simulink model "q2_sim_pid"  (R2019b)
settings: Solver=VariableStepAuto  StartTime=0.0  StopTime=50  RelTol=1e-3
libraries: simulink x2
settings Model: Creator=Mertcan  LastModifiedBy=Mertcan

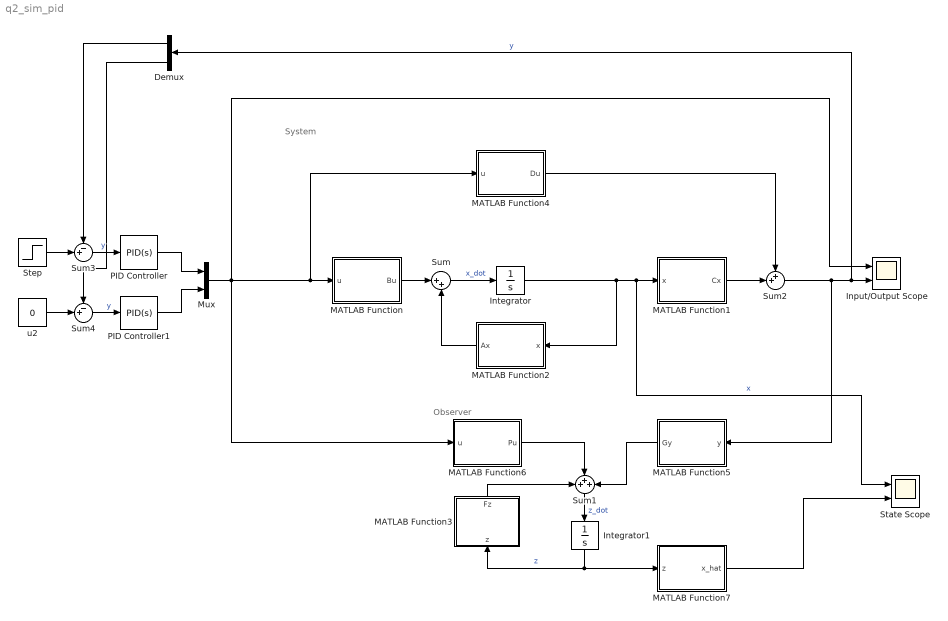
== system q2_sim_pid ==
  note: Observer
  note: System
  Demux : Demux  Outputs=2
  Input/Output Scope : Scope  NumInputPorts=2
  Integrator : Integrator
  Integrator1 : Integrator
  MATLAB Function : MATLAB Function  TreatAsAtomicUnit=on
  MATLAB Function1 : MATLAB Function  TreatAsAtomicUnit=on
  MATLAB Function2 : MATLAB Function  TreatAsAtomicUnit=on
  MATLAB Function3 : MATLAB Function  TreatAsAtomicUnit=on
  MATLAB Function4 : MATLAB Function  TreatAsAtomicUnit=on
  MATLAB Function5 : MATLAB Function  TreatAsAtomicUnit=on
  MATLAB Function6 : MATLAB Function  TreatAsAtomicUnit=on
  MATLAB Function7 : MATLAB Function  TreatAsAtomicUnit=on
  Mux : Mux  Inputs=2
  PID Controller : simulink/Continuous/PID Controller  Controller=PID  Form=Parallel  TimeDomain=Continuous-time  SampleTime=-1  IntegratorMethod=Forward Euler  FilterMethod=Forward Euler  ControllerParametersSource=internal  P=1  I=1  D=0  UseFilter=on  N=100  TunerSelectOption=Transfer Function Based (PID Tuner App)  InitialConditionSource=internal  InitialConditionForIntegrator=0  InitialConditionForFilter=0  DifferentiatorICPrevScaledInput=0  ExternalReset=none  TrackingMode=off  Kt=1  LimitOutput=off  UpperSaturationLimit=inf  LowerSaturationLimit=-inf  LinearizeAsGain=on  AntiWindupMode=none  Kb=1  POutMin=[]  POutMax=[]  IOutMin=[]  IOutMax=[]  DOutMin=[]  DOutMax=[]  NOutMin=[]  NOutMax=[]  SumOutMin=[]  SumOutMax=[]  SaturationOutMin=[]  SaturationOutMax=[]  PParamMin=[]  PParamMax=[]  IParamMin=[]  IParamMax=[]  DParamMin=[]  DParamMax=[]  NParamMin=[]  NParamMax=[]  KbParamMin=[]  KbParamMax=[]  KtParamMin=[]  KtParamMax=[]  KbOutMin=[]  KbOutMax=[]  KtOutMin=[]  KtOutMax=[]  IntegratorOutMin=[]  IntegratorOutMax=[]  FilterOutMin=[]  FilterOutMax=[]  SumI1OutMin=[]  SumI1OutMax=[]  SumI2OutMin=[]  SumI2OutMax=[]  SumI3OutMin=[]  SumI3OutMax=[]  SumI4OutMin=[]  SumI4OutMax=[]  SumDOutMin=[]  SumDOutMax=[]  DifferentiatorOutMin=[]  DifferentiatorOutMax=[]  FilterDiffOutCoefMin=[]  FilterDiffOutCoefMax=[]  ReciprocalOutMin=[]  ReciprocalOutMax=[]  SumDenOutMin=[]  SumDenOutMax=[]  SumNumOutMin=[]  SumNumOutMax=[]  DivideOutMin=[]  DivideOutMax=[]  IntegratorContinuousStateAttributes=''  IntegratorStateMustResolveToSignalObject=off  IntegratorRTWStateStorageClass=Auto  FilterContinuousStateAttributes=''  FilterStateMustResolveToSignalObject=off  FilterRTWStateStorageClass=Auto  ParallelPVariant=InternalParameters  IdealPVariant=Disabled  IVariant=InternalParameters  DVariant=InternalParameters  IntegratorVariant=Continuous  SatVariant=Disabled  AWVariant=Passthrough  PCopyVariant=Disabled  TRVariant=Disabled  FdbkBlocksVariant=Forward  IdealPFdbkVariant=Disabled  SatFdbkVariant=Disabled  DerivativeFilterVariant=ContFilter  NVariant=InternalParameters  NCopyVariant=Disabled  FilterICVariant=InternalICsFilter  IntegratorICVariant=InternalICs  ExternalResetVariant=Disabled  TRSumVariant=Passthrough  SumFdbkVariant=Disabled  SumVariant=Sum_PID
  PID Controller1 : simulink/Continuous/PID Controller  Controller=PID  Form=Parallel  TimeDomain=Continuous-time  SampleTime=-1  IntegratorMethod=Forward Euler  FilterMethod=Forward Euler  ControllerParametersSource=internal  P=1  I=1  D=0  UseFilter=on  N=100  TunerSelectOption=Transfer Function Based (PID Tuner App)  InitialConditionSource=internal  InitialConditionForIntegrator=0  InitialConditionForFilter=0  DifferentiatorICPrevScaledInput=0  ExternalReset=none  TrackingMode=off  Kt=1  LimitOutput=off  UpperSaturationLimit=inf  LowerSaturationLimit=-inf  LinearizeAsGain=on  AntiWindupMode=none  Kb=1  POutMin=[]  POutMax=[]  IOutMin=[]  IOutMax=[]  DOutMin=[]  DOutMax=[]  NOutMin=[]  NOutMax=[]  SumOutMin=[]  SumOutMax=[]  SaturationOutMin=[]  SaturationOutMax=[]  PParamMin=[]  PParamMax=[]  IParamMin=[]  IParamMax=[]  DParamMin=[]  DParamMax=[]  NParamMin=[]  NParamMax=[]  KbParamMin=[]  KbParamMax=[]  KtParamMin=[]  KtParamMax=[]  KbOutMin=[]  KbOutMax=[]  KtOutMin=[]  KtOutMax=[]  IntegratorOutMin=[]  IntegratorOutMax=[]  FilterOutMin=[]  FilterOutMax=[]  SumI1OutMin=[]  SumI1OutMax=[]  SumI2OutMin=[]  SumI2OutMax=[]  SumI3OutMin=[]  SumI3OutMax=[]  SumI4OutMin=[]  SumI4OutMax=[]  SumDOutMin=[]  SumDOutMax=[]  DifferentiatorOutMin=[]  DifferentiatorOutMax=[]  FilterDiffOutCoefMin=[]  FilterDiffOutCoefMax=[]  ReciprocalOutMin=[]  ReciprocalOutMax=[]  SumDenOutMin=[]  SumDenOutMax=[]  SumNumOutMin=[]  SumNumOutMax=[]  DivideOutMin=[]  DivideOutMax=[]  IntegratorContinuousStateAttributes=''  IntegratorStateMustResolveToSignalObject=off  IntegratorRTWStateStorageClass=Auto  FilterContinuousStateAttributes=''  FilterStateMustResolveToSignalObject=off  FilterRTWStateStorageClass=Auto  ParallelPVariant=InternalParameters  IdealPVariant=Disabled  IVariant=InternalParameters  DVariant=InternalParameters  IntegratorVariant=Continuous  SatVariant=Disabled  AWVariant=Passthrough  PCopyVariant=Disabled  TRVariant=Disabled  FdbkBlocksVariant=Forward  IdealPFdbkVariant=Disabled  SatFdbkVariant=Disabled  DerivativeFilterVariant=ContFilter  NVariant=InternalParameters  NCopyVariant=Disabled  FilterICVariant=InternalICsFilter  IntegratorICVariant=InternalICs  ExternalResetVariant=Disabled  TRSumVariant=Passthrough  SumFdbkVariant=Disabled  SumVariant=Sum_PID
  State Scope : Scope  NumInputPorts=2
  Step : Step  SampleTime=0
  Sum : Sum  Inputs=|++
  Sum1 : Sum  Inputs=+++
  Sum2 : Sum  Inputs=++|
  Sum3 : Sum  Inputs=-+|
  Sum4 : Sum  Inputs=-+|
  u2 : Constant  Value=0
  wires:
  MATLAB Function/1(Bu) -> Sum/1
  Sum/1 -> Integrator/1  "x_dot"
  MATLAB Function2/1(Ax) -> Sum/2
  MATLAB Function1/1(Cx) -> Sum2/2
  MATLAB Function4/1(Du) -> Sum2/1
  Sum2/1 -> MATLAB Function5/1(y), Demux/1, Input/Output Scope/2  "y"
  Integrator/1 -> State Scope/1, MATLAB Function1/1(x), MATLAB Function2/1(x)  "x"
  Sum1/1 -> Integrator1/1  "z_dot"
  Integrator1/1 -> MATLAB Function3/1(z), MATLAB Function7/1(z)  "z"
  MATLAB Function5/1(Gy) -> Sum1/3
  MATLAB Function6/1(Pu) -> Sum1/2
  MATLAB Function3/1(Fz) -> Sum1/1
  MATLAB Function7/1(x_hat) -> State Scope/2
  Mux/1 -> Input/Output Scope/1, MATLAB Function6/1(u), MATLAB Function4/1(u), MATLAB Function/1(u)
  Step/1 -> Sum3/2
  Sum3/1 -> PID Controller/1  "y"
  PID Controller/1 -> Mux/1
  Sum4/1 -> PID Controller1/1  "y"
  u2/1 -> Sum4/2
  PID Controller1/1 -> Mux/2
  Demux/2 -> Sum4/1
  Demux/1 -> Sum3/1

== matlab function q2_sim_pid/MATLAB Function1 ==
  data: x input; Cx output
function Cx = Cmat(x)

C = [0, 1, 0, 0
    0, 0, 0, 57.3];

Cx = C*x;

== matlab function q2_sim_pid/MATLAB Function ==
  data: u input; Bu output
function Bu = Bmat(u)

B = [0.14, -0.12
    0.36, -8.6
    0.35, 0.009
    0, 0];

Bu = B*u;

== matlab function q2_sim_pid/MATLAB Function2 ==
  data: x input; Ax output
function Ax = Amat(x)

A = [-0.02, 0.005, 2.4, -32
    -0.14, 0.44, -1.3, -30
    0, 0.018, -1.6, 1.2
    0, 0, 1, 0];

Ax = A*x;

== matlab function q2_sim_pid/MATLAB Function3 ==
  data: z input; Fz output
function Fz = Fmat(z)

F = [-1, 0, 0, 0
    0, -2, 0, 0
    0, 0, -3, 0
    0, 0, 0, -4];

Fz = F*z;

== matlab function q2_sim_pid/MATLAB Function4 ==
  data: u input; Du output
function Du = Dmat(u)

D = [0 0
    0 0];

Du = D*u;

== matlab function q2_sim_pid/MATLAB Function5 ==
  data: y input; Gy output
function Gy = Gmat(y)

G = [1, 2
    2, 3
    3, 4
    4, 5];

Gy = G*y;

== matlab function q2_sim_pid/MATLAB Function6 ==
  data: u input; Pu output
function Pu = Pmat(u)

P = [21.7151, 1.26724
 110.13, 15.8722
 -30.6081, -12.3048
 -12.7052, -9.39228];
 
Pu = P*u;

== matlab function q2_sim_pid/MATLAB Function7 ==
  data: z input; x_hat output
function x_hat = invXmat(z)

invX = [-37.8567, 32.7562, 153.738, -151.151
 -1.17795, -0.116633, -3.28679, 4.86561
 -0.00801532, 0.0105963, 0.0316064, -0.02554
 0.0257213, -0.00761971, -0.0115383, 0.00570989];
 
x_hat = invX*z;
